simulink model "CtrPlatform"  (Simulink 7.9)
settings: Solver=ode3  StartTime=0.0  StopTime=8  FixedStep=Ts  RelTol=1e-3
InitFcn:
  | eval('CtrPlatformCfg')
StopFcn:
  | eval('CtrPlotTrj')
values from neighbouring files (symbols this model uses):
  A = [a1 a2 a3 a4 a5 a6]/180*pi    [Config.m]    (also in CtrPlatformCfg.m)
  a2 = 0    [Config.m]    (also in CtrPlatformCfg.m)
  a3 = 0    [Config.m]    (also in CtrPlatformCfg.m)
  a4 = 0    [Config.m]    (also in CtrPlatformCfg.m)
  a5 = 90    [Config.m]    (also in CtrPlatformCfg.m)
  a6 = 0    [Config.m]    (also in CtrPlatformCfg.m)
  Cen = Cen(:)'    [Config.m]    (also in CtrPlatformCfg.m; DynEulerTest.m = Cen'; EfDynCAD.m = [cen1,cen2,cen3,cen4,cen5,cen6]')
  CurPulseFreq = 0.25*2*pi    (= 1.57079632679)    [Config.m]    (also in CtrPlatformCfg.m)
  Deg2Rad = pi/180    (= 0.0174532925199)    [Config.m]    (also in CtrPlatformCfg.m)
  DisturbSelect = 2    [Config.m]    (also in CtrPlatformCfg.m)
  DynTrjMode = 3    [Config.m]    (also in CtrPlatformCfg.m = 1)
  FbDisturbSelect = 2    [Config.m]    (also in CtrPlatformCfg.m)
  freq = tvel/radius    (= 1)    [Config.m]    (also in CtrPlatformCfg.m)
  FrictionSelect = 2    [CtrPlatformCfg.m]
  Gravity = 9.8    [Config.m]    (also in CtrPlatformCfg.m)
  Ie1 = in1(:)'    [Config.m]    (also in CtrPlatformCfg.m; DynEulerTest.m = in1(:); EfDynCAD.m = in1(:))
  Ie2 = in2(:)'    [Config.m]    (also in CtrPlatformCfg.m; DynEulerTest.m = in2(:); EfDynCAD.m = in2(:))
  Ie3 = in3(:)'    [Config.m]    (also in CtrPlatformCfg.m; DynEulerTest.m = in3(:); EfDynCAD.m = in3(:))
  Ie4 = in4(:)'    [Config.m]    (also in CtrPlatformCfg.m; DynEulerTest.m = in4(:); EfDynCAD.m = in4(:))
  Ie5 = in5(:)'    [Config.m]    (also in CtrPlatformCfg.m; DynEulerTest.m = in5(:); EfDynCAD.m = in5(:))
  Ie6 = in6(:)'    [Config.m]    (also in CtrPlatformCfg.m; DynEulerTest.m = in6(:); EfDynCAD.m = in6(:))
  in1 = [5.2954 -0.2565 -0.6366;-0.2565 4.7000 0.2830;-0.6366 0.2829 5.8635]    [Config.m]    (also in CtrPlatformCfg.m; DynEulerTest.m; EfDynCAD.m = [0.54  -0.01 0.23)
  in2 = [5.8840 0.0072 0.0135;0.0072 6.0178 -0.1907;0.0135 -0.1907 0.3374]    [Config.m]    (also in CtrPlatformCfg.m; DynEulerTest.m; EfDynCAD.m = (R_x*R_z)*in2*(R_x*R_z)')
  in3 = [1.8201 -0.2274 -0.3112;-0.2274 2.2537 -0.1441;-0.3112 -0.1441 1.9485]    [Config.m]    (also in CtrPlatformCfg.m; DynEulerTest.m; EfDynCAD.m = (R_x*R_z)*in3*(R_x*R_z)')
  in4 = [0.0607 -0.0922 0;-0.0922 1.4493 0;0 0 1.4620]    [Config.m]    (also in CtrPlatformCfg.m; DynEulerTest.m = [0.0607 -0.0922 0;-0.0922 1.4493 0;0 0,1.4620]; EfDynCAD.m = (R_y*Rz)*in4*(R_y*Rz)')
  in5 = [0.0191 0.0032 0;0.0032 0.0228 0;0 0 0.0291]    [Config.m]    (also in CtrPlatformCfg.m; DynEulerTest.m; EfDynCAD.m = (R_x*R_y)*in5*(R_x*R_y)')
  in6 = [0.0012 0 0;0 0.0007 0;0 0 0.0007]    [Config.m]    (also in CtrPlatformCfg.m; DynEulerTest.m; EfDynCAD.m = (R_y*Rz)*in6*(R_y*Rz)')
  init_Endx = gd_init(1,4)    [Config.m]    (also in CtrPlatformCfg.m)
  init_Endy = gd_init(2,4)    [Config.m]    (also in CtrPlatformCfg.m)
  init_Endz = gd_init(3,4)    [Config.m]    (also in CtrPlatformCfg.m)
  init_Rot = gd_init(1:3,1:3)    [Config.m]    (also in CtrPlatformCfg.m)
  JntOffset1 = A(1)    [Config.m]    (also in CtrPlatformCfg.m)
  JntOffset2 = A(2)    [Config.m]    (also in CtrPlatformCfg.m)
  JntOffset3 = A(3)    [Config.m]    (also in CtrPlatformCfg.m)
  JntOffset4 = A(4)    [Config.m]    (also in CtrPlatformCfg.m)
  JntOffset5 = A(5)    [Config.m]    (also in CtrPlatformCfg.m)
  JntOffset6 = A(6)    [Config.m]    (also in CtrPlatformCfg.m)
  L = [l1 l2 l3 l4 l5 l6 l7 l8 l9]    [Config.m]    (also in CtrPlatformCfg.m)
  LinePTs2RadpS = 2*pi/(EncRes*Ts)./Gear    [Config.m]    (also in CtrPlatformCfg.m)
  LinePTs2Rpm = 60/(EncRes*Ts)    (= 7.32421875)    [Config.m]    (also in CtrPlatformCfg.m)
  Ma = [ma1 ma2 ma3 ma4 ma5 ma6]    [Config.m]    (also in CtrPlatformCfg.m; DynEulerTest.m = [ma1; ma2; ma3; ma4; ma5; ma6]; EfDynCAD.m = [ma1 ma2 ma3 ma4 ma5 ma6]')
  ma1 = 170.31    [Config.m]    (also in CtrPlatformCfg.m; DynEulerTest.m; EfDynCAD.m = 77.75)
  ma2 = 63.74    [Config.m]    (also in CtrPlatformCfg.m; DynEulerTest.m; EfDynCAD.m = 32.31)
  ma3 = 98.98    [Config.m]    (also in CtrPlatformCfg.m; DynEulerTest.m; EfDynCAD.m = 18.61)
  ma4 = 24.46    [Config.m]    (also in CtrPlatformCfg.m; DynEulerTest.m; EfDynCAD.m = 15.65)
  ma5 = 5.24    [Config.m]    (also in CtrPlatformCfg.m; DynEulerTest.m; EfDynCAD.m = 3.32)
  ma6 = 0.6    [Config.m]    (also in CtrPlatformCfg.m; DynEulerTest.m; EfDynCAD.m)
  PosPulseEnable = 1    [Config.m]    (also in CtrPlatformCfg.m)
  PosVelPulseGain = 500    [Config.m]    (also in CtrPlatformCfg.m)
  Rad2Line = Gear*EncRes/(2*pi)    [Config.m]    (also in CtrPlatformCfg.m)
  Rpm2LinePTs = EncRes*Ts/60    (= 0.136533333333)    [Config.m]    (also in CtrPlatformCfg.m)
  TrajSwitch = 1    [Config.m]    (also in CtrPlatformCfg.m)
  Trq2Cur = Trq2Cur./Cur2Trq    [Config.m]    (also in CtrPlatformCfg.m)
  Ts = 1/FrHz    (= 0.00025)    [Config.m]    (also in CtrPlatformCfg.m)
  Ts_Dyn = Ts    (= 0.00025)    [Config.m]    (also in CtrPlatformCfg.m)
  tvel = 120    [Config.m]    (also in CtrPlatformCfg.m)
  VelLpAxisNum = 1    [Config.m]    (also in CtrPlatformCfg.m)
  VelPulseEnable = 0    [Config.m]    (also in CtrPlatformCfg.m)
  VelPulseGain = 500    [Config.m]    (also in CtrPlatformCfg.m)
  Volt2Trq = Volt2Trq./Trq2Cur    [Config.m]    (also in CtrPlatformCfg.m)
undefined symbols (not defined in the file or in its folder): a1, DiscIntNeverNeededParam, RobotAxis
libraries: simulink x85, mblibv1 x35, powerlib_extras x25, commnoisgen2 x2
(part 3 of 5)

== system CtrPlatform/Trajectory Generator/Circle in Descartes Space ==
  Difference{,1..3} (4 alike) : simulink/Discrete/Difference  ICPrevInput=0.0  InputProcessing=Inherited  OutMin=[]  OutMax=[]  OutDataType=fixdt(1, 16)  OutScaling=2^-10  DoSatur=off
  Discrete-Time Integrator : DiscreteIntegrator  InitialCondition=init_Endx  SampleTime=Ts_Dyn  ICPrevOutput=DiscIntNeverNeededParam  ICPrevScaledInput=DiscIntNeverNeededParam
  Discrete-Time Integrator1 : DiscreteIntegrator  InitialCondition=init_Endy  SampleTime=Ts_Dyn  ICPrevOutput=DiscIntNeverNeededParam  ICPrevScaledInput=DiscIntNeverNeededParam
  Discrete-Time Integrator2 : DiscreteIntegrator  InitialCondition=init_Endz  SampleTime=Ts_Dyn  ICPrevOutput=DiscIntNeverNeededParam  ICPrevScaledInput=DiscIntNeverNeededParam
  EndVelocity : Subsystem
  Inverse Kinematic : MATLAB Function  TreatAsAtomicUnit=on
  Jacobian : MATLAB Function  TreatAsAtomicUnit=on
  Mux{1..3,5..6} (5 alike) : Mux  Inputs=3
  Mux4 : Mux  Inputs=5
  Rad2Deg : Gain  Gain=180/pi
  "Re-group " : Subsystem
  Zero : Gain  Gain=0
  Zero1 : Gain  Gain=1/Ts_Dyn
  Zero2 : Gain  Gain=1/Ts_Dyn
  Ref_JJVVAA : Outport
  RefEnd : Outport  Port=2
  Ref_JVAJVA : Outport  Port=3
  wires:
  Discrete-Time Integrator/1 -> Mux2/1
  Discrete-Time Integrator1/1 -> Mux2/2
  EndVelocity/1(EndVx) -> Mux1/1, Mux5/1, Difference/1, Discrete-Time Integrator/1
  EndVelocity/2(EndVy) -> Mux1/2, Mux5/2, Difference1/1, Discrete-Time Integrator1/1
  EndVelocity/3(EndVz) -> Mux1/3, Mux5/3, Difference2/1, Discrete-Time Integrator2/1
  Discrete-Time Integrator2/1 -> Mux2/3
  Mux2/1 -> Inverse Kinematic/1(EndPos), Mux4/1
  Inverse Kinematic/1(Theta) -> Jacobian/1(Theta), Mux3/1
  Mux4/1 -> RefEnd/1
  Difference/1 -> Mux6/1
  Difference1/1 -> Mux6/2
  Difference2/1 -> Mux6/3
  Mux1/1 -> Jacobian/2(EndVel)
  Jacobian/1(Omega) -> Mux3/2, Difference3/1
  Difference3/1 -> Zero2/1
  Mux3/1 -> Ref_JJVVAA/1, "Re-group "/1(JJVVAA)
  "Re-group "/1(JVAJVA) -> Rad2Deg/1
  Mux5/1 -> Mux4/2
  Mux6/1 -> Zero1/1
  Zero/1 -> Mux4/3, Mux4/5
  Rad2Deg/1 -> Ref_JVAJVA/1
  Zero1/1 -> Mux4/4, Zero/1
  Zero2/1 -> Mux3/3

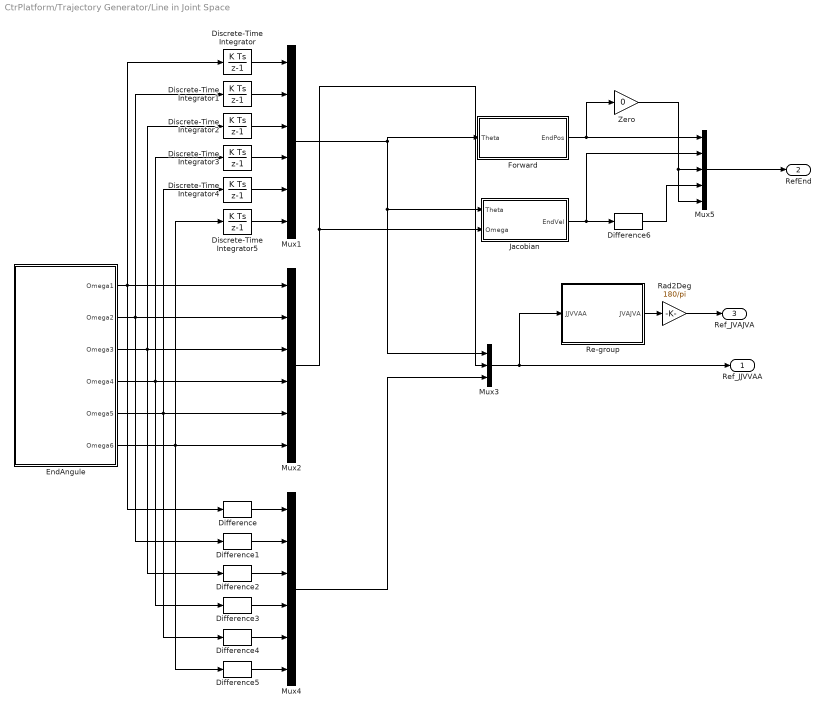
== system CtrPlatform/Trajectory Generator/Line in Joint Space ==
  Difference{,1..6} (7 alike) : simulink/Discrete/Difference  ICPrevInput=0.0  InputProcessing=Inherited  OutMin=[]  OutMax=[]  OutDataType=fixdt(1, 16)  OutScaling=2^-10  DoSatur=off
  Discrete-Time Integrator : DiscreteIntegrator  InitialCondition=a1/180*pi  SampleTime=Ts_Dyn  ICPrevOutput=DiscIntNeverNeededParam  ICPrevScaledInput=DiscIntNeverNeededParam
  Discrete-Time Integrator1 : DiscreteIntegrator  InitialCondition=a2/180*pi  SampleTime=Ts_Dyn  ICPrevOutput=DiscIntNeverNeededParam  ICPrevScaledInput=DiscIntNeverNeededParam
  Discrete-Time Integrator2 : DiscreteIntegrator  InitialCondition=a3/180*pi  SampleTime=Ts_Dyn  ICPrevOutput=DiscIntNeverNeededParam  ICPrevScaledInput=DiscIntNeverNeededParam
  Discrete-Time Integrator3 : DiscreteIntegrator  InitialCondition=a4/180*pi  SampleTime=Ts_Dyn  ICPrevOutput=DiscIntNeverNeededParam  ICPrevScaledInput=DiscIntNeverNeededParam
  Discrete-Time Integrator4 : DiscreteIntegrator  InitialCondition=a5/180*pi  SampleTime=Ts_Dyn  ICPrevOutput=DiscIntNeverNeededParam  ICPrevScaledInput=DiscIntNeverNeededParam
  Discrete-Time Integrator5 : DiscreteIntegrator  InitialCondition=a6/180*pi  SampleTime=Ts_Dyn  ICPrevOutput=DiscIntNeverNeededParam  ICPrevScaledInput=DiscIntNeverNeededParam
  EndAngule : Subsystem
  Forward : MATLAB Function  TreatAsAtomicUnit=on
  Jacobian : MATLAB Function  TreatAsAtomicUnit=on
  Mux1 : Mux  Inputs=6
  Mux2 : Mux  Inputs=6
  Mux3 : Mux  Inputs=3
  Mux4 : Mux  Inputs=6
  Mux5 : Mux  Inputs=5
  Rad2Deg : Gain  Gain=180/pi
  "Re-group " : Subsystem
  Zero : Gain  Gain=0
  Ref_JJVVAA : Outport
  RefEnd : Outport  Port=2
  Ref_JVAJVA : Outport  Port=3
  wires:
  Forward/1(EndPos) -> Mux5/1, Zero/1
  Mux5/1 -> RefEnd/1
  Mux4/1 -> Mux3/3
  Mux1/1 -> Jacobian/1(Theta), Mux3/1, Forward/1(Theta)
  Mux2/1 -> Jacobian/2(Omega), Mux3/2
  Difference5/1 -> Mux4/6
  Difference4/1 -> Mux4/5
  Difference3/1 -> Mux4/4
  Difference2/1 -> Mux4/3
  Difference1/1 -> Mux4/2
  Difference/1 -> Mux4/1
  Discrete-Time Integrator5/1 -> Mux1/6
  Discrete-Time Integrator4/1 -> Mux1/5
  Discrete-Time Integrator3/1 -> Mux1/4
  Discrete-Time Integrator2/1 -> Mux1/3
  Discrete-Time Integrator1/1 -> Mux1/2
  Discrete-Time Integrator/1 -> Mux1/1
  EndAngule/6(Omega6) -> Mux2/6, Discrete-Time Integrator5/1, Difference5/1
  EndAngule/5(Omega5) -> Mux2/5, Discrete-Time Integrator4/1, Difference4/1
  EndAngule/4(Omega4) -> Mux2/4, Discrete-Time Integrator3/1, Difference3/1
  EndAngule/3(Omega3) -> Mux2/3, Discrete-Time Integrator2/1, Difference2/1
  EndAngule/2(Omega2) -> Mux2/2, Discrete-Time Integrator1/1, Difference1/1
  EndAngule/1(Omega1) -> Mux2/1, Discrete-Time Integrator/1, Difference/1
  Mux3/1 -> Ref_JJVVAA/1, "Re-group "/1(JJVVAA)
  "Re-group "/1(JVAJVA) -> Rad2Deg/1
  Jacobian/1(EndVel) -> Mux5/2, Difference6/1
  Difference6/1 -> Mux5/4
  Zero/1 -> Mux5/3, Mux5/5
  Rad2Deg/1 -> Ref_JVAJVA/1

== system CtrPlatform/Trajectory Generator/Still ==
  Difference{,1..3} (4 alike) : simulink/Discrete/Difference  ICPrevInput=0.0  InputProcessing=Inherited  OutMin=[]  OutMax=[]  OutDataType=fixdt(1, 16)  OutScaling=2^-10  DoSatur=off
  Discrete-Time Integrator : DiscreteIntegrator  InitialCondition=init_Endx  SampleTime=Ts_Dyn  ICPrevOutput=DiscIntNeverNeededParam  ICPrevScaledInput=DiscIntNeverNeededParam
  Discrete-Time Integrator1 : DiscreteIntegrator  InitialCondition=init_Endy  SampleTime=Ts_Dyn  ICPrevOutput=DiscIntNeverNeededParam  ICPrevScaledInput=DiscIntNeverNeededParam
  Discrete-Time Integrator2 : DiscreteIntegrator  InitialCondition=init_Endz  SampleTime=Ts_Dyn  ICPrevOutput=DiscIntNeverNeededParam  ICPrevScaledInput=DiscIntNeverNeededParam
  EndVelocity : Subsystem
  Inverse Kinematic : MATLAB Function  TreatAsAtomicUnit=on
  Jacobian : MATLAB Function  TreatAsAtomicUnit=on
  Mux{1..3,5..6} (5 alike) : Mux  Inputs=3
  Mux4 : Mux  Inputs=5
  Rad2Deg : Gain  Gain=180/pi
  "Re-group " : Subsystem
  Zero : Gain  Gain=0
  Ref_JJVVAA : Outport
  RefEnd : Outport  Port=2
  Ref_JVAJVA : Outport  Port=3
  wires:
  Zero/1 -> Mux4/5, Mux4/3
  Mux6/1 -> Zero/1, Mux4/4
  Mux5/1 -> Mux4/2
  "Re-group "/1(JVAJVA) -> Rad2Deg/1
  Mux3/1 -> "Re-group "/1(JJVVAA), Ref_JJVVAA/1
  Difference3/1 -> Mux3/3
  Jacobian/1(Omega) -> Mux3/2, Difference3/1
  Mux1/1 -> Jacobian/2(EndVel)
  Difference2/1 -> Mux6/3
  Difference1/1 -> Mux6/2
  Difference/1 -> Mux6/1
  Mux4/1 -> RefEnd/1
  Inverse Kinematic/1(Theta) -> Mux3/1, Jacobian/1(Theta)
  Mux2/1 -> Mux4/1, Inverse Kinematic/1(EndPos)
  Discrete-Time Integrator2/1 -> Mux2/3
  EndVelocity/3(EndVz) -> Mux5/3, Difference2/1, Mux1/3, Discrete-Time Integrator2/1
  EndVelocity/2(EndVy) -> Mux5/2, Difference1/1, Mux1/2, Discrete-Time Integrator1/1
  EndVelocity/1(EndVx) -> Mux5/1, Difference/1, Mux1/1, Discrete-Time Integrator/1
  Discrete-Time Integrator1/1 -> Mux2/2
  Discrete-Time Integrator/1 -> Mux2/1
  Rad2Deg/1 -> Ref_JVAJVA/1

== system CtrPlatform/Controller/Controller Axis 1/EncDiff2Vel(LpTs) ==
  Enc : Inport
  Add : Sum  Inputs=+-
  Discrete  2nd-Order Filter : powerlib_extras/Discrete  Control Blocks/Discrete  2nd-Order Filter  FilterType=Lowpass  Fo=200  Zeta=0.707  Ts=Ts  Initialize=off  Vac_Init=[0.8 -25 60]  Vdc_Init=-0.4  PlotResponse=off  param1=[1 5000 10]
  EncVel(rpm) : Scope
      settings: SaveName=ScopeData33
  Integer Delay : Delay  DelayLength=1  InitialCondition=0  InputProcessing=Inherited
  LinePTs2Rpm : Gain  Gain=LinePTs2Rpm
  Vel : Outport
  wires:
  LinePTs2Rpm/1 -> EncVel(rpm)/1
  Integer Delay/1 -> Add/2
  Enc/1 -> Add/1, Integer Delay/1
  Discrete  2nd-Order Filter/1 -> LinePTs2Rpm/1, Vel/1
  Add/1 -> Discrete  2nd-Order Filter/1

== system CtrPlatform/Controller/Controller Axis 1/EncDiff2Vel(LpTs)1 ==
  Enc : Inport
  Add : Sum  Inputs=+-
  Discrete  2nd-Order Filter : powerlib_extras/Discrete  Control Blocks/Discrete  2nd-Order Filter  FilterType=Lowpass  Fo=200  Zeta=0.707  Ts=Ts  Initialize=off  Vac_Init=[0.8 -25 60]  Vdc_Init=-0.4  PlotResponse=off  param1=[1 5000 10]
  EncVel(rpm) : Scope
      settings: SaveName=ScopeData33
  Integer Delay : Delay  DelayLength=1  InitialCondition=0  InputProcessing=Inherited
  LinePTs2Rpm : Gain  Gain=LinePTs2Rpm
  Vel : Outport
  wires:
  Add/1 -> Discrete  2nd-Order Filter/1
  Discrete  2nd-Order Filter/1 -> Vel/1, LinePTs2Rpm/1
  Enc/1 -> Integer Delay/1, Add/1
  Integer Delay/1 -> Add/2
  LinePTs2Rpm/1 -> EncVel(rpm)/1

== system CtrPlatform/Controller/Controller Axis 1/Error Check and Lock Error ==
  PositionCheck(Line) : Inport
  VelocityCheck(LpTs) : Inport  Port=2
  Abs : Abs
  Abs1 : Abs
  Compare To Constant : simulink/Logic and Bit Operations/Compare To Constant  relop=<=  const=VelErrorCheckLimit  OutDataTypeStr=uint8  ZeroCross=off
  Compare To Constant1 : simulink/Logic and Bit Operations/Compare To Constant  relop=<=  const=PosErrorCheckLimit  OutDataTypeStr=uint8  ZeroCross=off
  Logical Operator : Logic  Inputs=3  AllPortsSameDT=off  OutDataTypeStr=boolean
  Unit Delay : UnitDelay  X0=1  SampleTime=Ts
  ErrorFlag : Outport
  wires:
  Logical Operator/1 -> Unit Delay/1, ErrorFlag/1
  Compare To Constant/1 -> Logical Operator/2
  Compare To Constant1/1 -> Logical Operator/1
  Abs1/1 -> Compare To Constant1/1
  Abs/1 -> Compare To Constant/1
  Unit Delay/1 -> Logical Operator/3
  PositionCheck(Line)/1 -> Abs1/1
  VelocityCheck(LpTs)/1 -> Abs/1

== system CtrPlatform/Controller/Controller Axis 1/IncPos(Line) ==
  Pos : Inport
  Add : Sum  Inputs=+-
  Int : DiscreteTransferFcn  Numerator=[1 0]  Denominator=[1 -1]  SampleTime=Ts
  Integer Delay : Delay  DelayLength=1  InitialCondition=InitialPos  InputProcessing=Inherited
  IncPos : Outport
  wires:
  Add/1 -> Int/1
  Pos/1 -> Add/1, Integer Delay/1
  Int/1 -> IncPos/1
  Integer Delay/1 -> Add/2

== system CtrPlatform/Controller/Controller Axis 1/Pos Controller ==
  Error(Line) : Inport
  Add1 : Sum  Inputs=+++
  D : Gain  Gain=Kd
  Diff : simulink/Discrete/Difference  ICPrevInput=0.0  InputProcessing=Inherited  OutMin=[]  OutMax=[]  OutDataType=sfix(16)  OutScaling=2^-10  DoSatur=off
  Discrete-Time Integrator : DiscreteIntegrator  SampleTime=Ts  ICPrevOutput=DiscIntNeverNeededParam  ICPrevScaledInput=DiscIntNeverNeededParam
  I : Gain  Gain=Ki
  p : Gain  Gain=Kp
  Vcmd(LpTs) : Outport
  wires:
  Diff/1 -> Add1/3
  Discrete-Time Integrator/1 -> Add1/2
  Add1/1 -> Vcmd(LpTs)/1
  Error(Line)/1 -> p/1, I/1, D/1
  p/1 -> Add1/1
  I/1 -> Discrete-Time Integrator/1
  D/1 -> Diff/1

== system CtrPlatform/Controller/Controller Axis 1/Vel Controller ==
  Error(LpTs) : Inport
  Add1 : Sum  Inputs=+++
  D : Gain  Gain=Kd
  Diff : simulink/Discrete/Difference  ICPrevInput=0.0  InputProcessing=Inherited  OutMin=[]  OutMax=[]  OutDataType=sfix(16)  OutScaling=2^-10  DoSatur=off
  Discrete-Time Integrator : DiscreteIntegrator  SampleTime=Ts  ICPrevOutput=DiscIntNeverNeededParam  ICPrevScaledInput=DiscIntNeverNeededParam
  I : Gain  Gain=Ki
  p : Gain  Gain=Kp
  Curcmd(Amp) : Outport
  wires:
  Discrete-Time Integrator/1 -> Add1/2
  Diff/1 -> Add1/3
  D/1 -> Diff/1
  Add1/1 -> Curcmd(Amp)/1
  I/1 -> Discrete-Time Integrator/1
  p/1 -> Add1/1
  Error(LpTs)/1 -> D/1, I/1, p/1

== system CtrPlatform/Controller/Controller Axis 2/EncDiff2Vel(LpTs) ==
  Enc : Inport
  Add : Sum  Inputs=+-
  Discrete  2nd-Order Filter : powerlib_extras/Discrete  Control Blocks/Discrete  2nd-Order Filter  FilterType=Lowpass  Fo=200  Zeta=0.707  Ts=Ts  Initialize=off  Vac_Init=[0.8 -25 60]  Vdc_Init=-0.4  PlotResponse=off  param1=[1 5000 10]
  EncVel(rpm) : Scope
      settings: SaveName=ScopeData33
  Integer Delay : Delay  DelayLength=1  InitialCondition=0  InputProcessing=Inherited
  LinePTs2Rpm : Gain  Gain=LinePTs2Rpm
  Vel : Outport
  wires:
  LinePTs2Rpm/1 -> EncVel(rpm)/1
  Integer Delay/1 -> Add/2
  Enc/1 -> Add/1, Integer Delay/1
  Discrete  2nd-Order Filter/1 -> LinePTs2Rpm/1, Vel/1
  Add/1 -> Discrete  2nd-Order Filter/1

== system CtrPlatform/Controller/Controller Axis 2/EncDiff2Vel(LpTs)1 ==
  Enc : Inport
  Add : Sum  Inputs=+-
  Discrete  2nd-Order Filter : powerlib_extras/Discrete  Control Blocks/Discrete  2nd-Order Filter  FilterType=Lowpass  Fo=200  Zeta=0.707  Ts=Ts  Initialize=off  Vac_Init=[0.8 -25 60]  Vdc_Init=-0.4  PlotResponse=off  param1=[1 5000 10]
  EncVel(rpm) : Scope
      settings: SaveName=ScopeData33
  Integer Delay : Delay  DelayLength=1  InitialCondition=0  InputProcessing=Inherited
  LinePTs2Rpm : Gain  Gain=LinePTs2Rpm
  Vel : Outport
  wires:
  Add/1 -> Discrete  2nd-Order Filter/1
  Discrete  2nd-Order Filter/1 -> Vel/1, LinePTs2Rpm/1
  Enc/1 -> Integer Delay/1, Add/1
  Integer Delay/1 -> Add/2
  LinePTs2Rpm/1 -> EncVel(rpm)/1

== system CtrPlatform/Controller/Controller Axis 2/Error Check and Lock Error ==
  PositionCheck(Line) : Inport
  VelocityCheck(LpTs) : Inport  Port=2
  Abs : Abs
  Abs1 : Abs
  Compare To Constant : simulink/Logic and Bit Operations/Compare To Constant  relop=<=  const=VelErrorCheckLimit  OutDataTypeStr=uint8  ZeroCross=off
  Compare To Constant1 : simulink/Logic and Bit Operations/Compare To Constant  relop=<=  const=PosErrorCheckLimit  OutDataTypeStr=uint8  ZeroCross=off
  Logical Operator : Logic  Inputs=3  AllPortsSameDT=off  OutDataTypeStr=boolean
  Unit Delay : UnitDelay  X0=1  SampleTime=Ts
  ErrorFlag : Outport
  wires:
  Logical Operator/1 -> Unit Delay/1, ErrorFlag/1
  Compare To Constant/1 -> Logical Operator/2
  Compare To Constant1/1 -> Logical Operator/1
  Abs1/1 -> Compare To Constant1/1
  Abs/1 -> Compare To Constant/1
  Unit Delay/1 -> Logical Operator/3
  PositionCheck(Line)/1 -> Abs1/1
  VelocityCheck(LpTs)/1 -> Abs/1

== system CtrPlatform/Controller/Controller Axis 2/IncPos(Line) ==
  Pos : Inport
  Add : Sum  Inputs=+-
  Int : DiscreteTransferFcn  Numerator=[1 0]  Denominator=[1 -1]  SampleTime=Ts
  Integer Delay : Delay  DelayLength=1  InitialCondition=InitialPos  InputProcessing=Inherited
  IncPos : Outport
  wires:
  Add/1 -> Int/1
  Pos/1 -> Add/1, Integer Delay/1
  Int/1 -> IncPos/1
  Integer Delay/1 -> Add/2

== system CtrPlatform/Controller/Controller Axis 2/Pos Controller ==
  Error(Line) : Inport
  Add1 : Sum  Inputs=+++
  D : Gain  Gain=Kd
  Diff : simulink/Discrete/Difference  ICPrevInput=0.0  InputProcessing=Inherited  OutMin=[]  OutMax=[]  OutDataType=sfix(16)  OutScaling=2^-10  DoSatur=off
  Discrete-Time Integrator : DiscreteIntegrator  SampleTime=Ts  ICPrevOutput=DiscIntNeverNeededParam  ICPrevScaledInput=DiscIntNeverNeededParam
  I : Gain  Gain=Ki
  p : Gain  Gain=Kp
  Vcmd(LpTs) : Outport
  wires:
  Diff/1 -> Add1/3
  Discrete-Time Integrator/1 -> Add1/2
  Add1/1 -> Vcmd(LpTs)/1
  Error(Line)/1 -> p/1, I/1, D/1
  p/1 -> Add1/1
  I/1 -> Discrete-Time Integrator/1
  D/1 -> Diff/1

== system CtrPlatform/Controller/Controller Axis 2/Vel Controller ==
  Error(LpTs) : Inport
  Add1 : Sum  Inputs=+++
  D : Gain  Gain=Kd
  Diff : simulink/Discrete/Difference  ICPrevInput=0.0  InputProcessing=Inherited  OutMin=[]  OutMax=[]  OutDataType=sfix(16)  OutScaling=2^-10  DoSatur=off
  Discrete-Time Integrator : DiscreteIntegrator  SampleTime=Ts  ICPrevOutput=DiscIntNeverNeededParam  ICPrevScaledInput=DiscIntNeverNeededParam
  I : Gain  Gain=Ki
  p : Gain  Gain=Kp
  Curcmd(Amp) : Outport
  wires:
  Discrete-Time Integrator/1 -> Add1/2
  Diff/1 -> Add1/3
  D/1 -> Diff/1
  Add1/1 -> Curcmd(Amp)/1
  I/1 -> Discrete-Time Integrator/1
  p/1 -> Add1/1
  Error(LpTs)/1 -> D/1, I/1, p/1

== system CtrPlatform/Controller/Controller Axis 3/EncDiff2Vel(LpTs) ==
  Enc : Inport
  Add : Sum  Inputs=+-
  Discrete  2nd-Order Filter : powerlib_extras/Discrete  Control Blocks/Discrete  2nd-Order Filter  FilterType=Lowpass  Fo=200  Zeta=0.707  Ts=Ts  Initialize=off  Vac_Init=[0.8 -25 60]  Vdc_Init=-0.4  PlotResponse=off  param1=[1 5000 10]
  EncVel(rpm) : Scope
      settings: SaveName=ScopeData33
  Integer Delay : Delay  DelayLength=1  InitialCondition=0  InputProcessing=Inherited
  LinePTs2Rpm : Gain  Gain=LinePTs2Rpm
  Vel : Outport
  wires:
  LinePTs2Rpm/1 -> EncVel(rpm)/1
  Integer Delay/1 -> Add/2
  Enc/1 -> Add/1, Integer Delay/1
  Discrete  2nd-Order Filter/1 -> LinePTs2Rpm/1, Vel/1
  Add/1 -> Discrete  2nd-Order Filter/1

== system CtrPlatform/Controller/Controller Axis 3/EncDiff2Vel(LpTs)1 ==
  Enc : Inport
  Add : Sum  Inputs=+-
  Discrete  2nd-Order Filter : powerlib_extras/Discrete  Control Blocks/Discrete  2nd-Order Filter  FilterType=Lowpass  Fo=200  Zeta=0.707  Ts=Ts  Initialize=off  Vac_Init=[0.8 -25 60]  Vdc_Init=-0.4  PlotResponse=off  param1=[1 5000 10]
  EncVel(rpm) : Scope
      settings: SaveName=ScopeData33
  Integer Delay : Delay  DelayLength=1  InitialCondition=0  InputProcessing=Inherited
  LinePTs2Rpm : Gain  Gain=LinePTs2Rpm
  Vel : Outport
  wires:
  Add/1 -> Discrete  2nd-Order Filter/1
  Discrete  2nd-Order Filter/1 -> Vel/1, LinePTs2Rpm/1
  Enc/1 -> Integer Delay/1, Add/1
  Integer Delay/1 -> Add/2
  LinePTs2Rpm/1 -> EncVel(rpm)/1

== system CtrPlatform/Controller/Controller Axis 3/Error Check and Lock Error ==
  PositionCheck(Line) : Inport
  VelocityCheck(LpTs) : Inport  Port=2
  Abs : Abs
  Abs1 : Abs
  Compare To Constant : simulink/Logic and Bit Operations/Compare To Constant  relop=<=  const=VelErrorCheckLimit  OutDataTypeStr=uint8  ZeroCross=off
  Compare To Constant1 : simulink/Logic and Bit Operations/Compare To Constant  relop=<=  const=PosErrorCheckLimit  OutDataTypeStr=uint8  ZeroCross=off
  Logical Operator : Logic  Inputs=3  AllPortsSameDT=off  OutDataTypeStr=boolean
  Unit Delay : UnitDelay  X0=1  SampleTime=Ts
  ErrorFlag : Outport
  wires:
  Logical Operator/1 -> Unit Delay/1, ErrorFlag/1
  Compare To Constant/1 -> Logical Operator/2
  Compare To Constant1/1 -> Logical Operator/1
  Abs1/1 -> Compare To Constant1/1
  Abs/1 -> Compare To Constant/1
  Unit Delay/1 -> Logical Operator/3
  PositionCheck(Line)/1 -> Abs1/1
  VelocityCheck(LpTs)/1 -> Abs/1

== system CtrPlatform/Controller/Controller Axis 3/IncPos(Line) ==
  Pos : Inport
  Add : Sum  Inputs=+-
  Int : DiscreteTransferFcn  Numerator=[1 0]  Denominator=[1 -1]  SampleTime=Ts
  Integer Delay : Delay  DelayLength=1  InitialCondition=InitialPos  InputProcessing=Inherited
  IncPos : Outport
  wires:
  Add/1 -> Int/1
  Pos/1 -> Add/1, Integer Delay/1
  Int/1 -> IncPos/1
  Integer Delay/1 -> Add/2

== system CtrPlatform/Controller/Controller Axis 3/Pos Controller ==
  Error(Line) : Inport
  Add1 : Sum  Inputs=+++
  D : Gain  Gain=Kd
  Diff : simulink/Discrete/Difference  ICPrevInput=0.0  InputProcessing=Inherited  OutMin=[]  OutMax=[]  OutDataType=sfix(16)  OutScaling=2^-10  DoSatur=off
  Discrete-Time Integrator : DiscreteIntegrator  SampleTime=Ts  ICPrevOutput=DiscIntNeverNeededParam  ICPrevScaledInput=DiscIntNeverNeededParam
  I : Gain  Gain=Ki
  p : Gain  Gain=Kp
  Vcmd(LpTs) : Outport
  wires:
  Diff/1 -> Add1/3
  Discrete-Time Integrator/1 -> Add1/2
  Add1/1 -> Vcmd(LpTs)/1
  Error(Line)/1 -> p/1, I/1, D/1
  p/1 -> Add1/1
  I/1 -> Discrete-Time Integrator/1
  D/1 -> Diff/1

== system CtrPlatform/Controller/Controller Axis 3/Vel Controller ==
  Error(LpTs) : Inport
  Add1 : Sum  Inputs=+++
  D : Gain  Gain=Kd
  Diff : simulink/Discrete/Difference  ICPrevInput=0.0  InputProcessing=Inherited  OutMin=[]  OutMax=[]  OutDataType=sfix(16)  OutScaling=2^-10  DoSatur=off
  Discrete-Time Integrator : DiscreteIntegrator  SampleTime=Ts  ICPrevOutput=DiscIntNeverNeededParam  ICPrevScaledInput=DiscIntNeverNeededParam
  I : Gain  Gain=Ki
  p : Gain  Gain=Kp
  Curcmd(Amp) : Outport
  wires:
  Discrete-Time Integrator/1 -> Add1/2
  Diff/1 -> Add1/3
  D/1 -> Diff/1
  Add1/1 -> Curcmd(Amp)/1
  I/1 -> Discrete-Time Integrator/1
  p/1 -> Add1/1
  Error(LpTs)/1 -> D/1, I/1, p/1

== system CtrPlatform/Controller/Controller Axis 4/EncDiff2Vel(LpTs) ==
  Enc : Inport
  Add : Sum  Inputs=+-
  Discrete  2nd-Order Filter : powerlib_extras/Discrete  Control Blocks/Discrete  2nd-Order Filter  FilterType=Lowpass  Fo=200  Zeta=0.707  Ts=Ts  Initialize=off  Vac_Init=[0.8 -25 60]  Vdc_Init=-0.4  PlotResponse=off  param1=[1 5000 10]
  EncVel(rpm) : Scope
      settings: SaveName=ScopeData33
  Integer Delay : Delay  DelayLength=1  InitialCondition=0  InputProcessing=Inherited
  LinePTs2Rpm : Gain  Gain=LinePTs2Rpm
  Vel : Outport
  wires:
  LinePTs2Rpm/1 -> EncVel(rpm)/1
  Integer Delay/1 -> Add/2
  Enc/1 -> Add/1, Integer Delay/1
  Discrete  2nd-Order Filter/1 -> LinePTs2Rpm/1, Vel/1
  Add/1 -> Discrete  2nd-Order Filter/1

== system CtrPlatform/Controller/Controller Axis 4/EncDiff2Vel(LpTs)1 ==
  Enc : Inport
  Add : Sum  Inputs=+-
  Discrete  2nd-Order Filter : powerlib_extras/Discrete  Control Blocks/Discrete  2nd-Order Filter  FilterType=Lowpass  Fo=200  Zeta=0.707  Ts=Ts  Initialize=off  Vac_Init=[0.8 -25 60]  Vdc_Init=-0.4  PlotResponse=off  param1=[1 5000 10]
  EncVel(rpm) : Scope
      settings: SaveName=ScopeData33
  Integer Delay : Delay  DelayLength=1  InitialCondition=0  InputProcessing=Inherited
  LinePTs2Rpm : Gain  Gain=LinePTs2Rpm
  Vel : Outport
  wires:
  Add/1 -> Discrete  2nd-Order Filter/1
  Discrete  2nd-Order Filter/1 -> Vel/1, LinePTs2Rpm/1
  Enc/1 -> Integer Delay/1, Add/1
  Integer Delay/1 -> Add/2
  LinePTs2Rpm/1 -> EncVel(rpm)/1

== system CtrPlatform/Controller/Controller Axis 4/Error Check and Lock Error ==
  PositionCheck(Line) : Inport
  VelocityCheck(LpTs) : Inport  Port=2
  Abs : Abs
  Abs1 : Abs
  Compare To Constant : simulink/Logic and Bit Operations/Compare To Constant  relop=<=  const=VelErrorCheckLimit  OutDataTypeStr=uint8  ZeroCross=off
  Compare To Constant1 : simulink/Logic and Bit Operations/Compare To Constant  relop=<=  const=PosErrorCheckLimit  OutDataTypeStr=uint8  ZeroCross=off
  Logical Operator : Logic  Inputs=3  AllPortsSameDT=off  OutDataTypeStr=boolean
  Unit Delay : UnitDelay  X0=1  SampleTime=Ts
  ErrorFlag : Outport
  wires:
  Logical Operator/1 -> Unit Delay/1, ErrorFlag/1
  Compare To Constant/1 -> Logical Operator/2
  Compare To Constant1/1 -> Logical Operator/1
  Abs1/1 -> Compare To Constant1/1
  Abs/1 -> Compare To Constant/1
  Unit Delay/1 -> Logical Operator/3
  PositionCheck(Line)/1 -> Abs1/1
  VelocityCheck(LpTs)/1 -> Abs/1

== system CtrPlatform/Controller/Controller Axis 4/IncPos(Line) ==
  Pos : Inport
  Add : Sum  Inputs=+-
  Int : DiscreteTransferFcn  Numerator=[1 0]  Denominator=[1 -1]  SampleTime=Ts
  Integer Delay : Delay  DelayLength=1  InitialCondition=InitialPos  InputProcessing=Inherited
  IncPos : Outport
  wires:
  Add/1 -> Int/1
  Pos/1 -> Add/1, Integer Delay/1
  Int/1 -> IncPos/1
  Integer Delay/1 -> Add/2

== system CtrPlatform/Controller/Controller Axis 4/Pos Controller ==
  Error(Line) : Inport
  Add1 : Sum  Inputs=+++
  D : Gain  Gain=Kd
  Diff : simulink/Discrete/Difference  ICPrevInput=0.0  InputProcessing=Inherited  OutMin=[]  OutMax=[]  OutDataType=sfix(16)  OutScaling=2^-10  DoSatur=off
  Discrete-Time Integrator : DiscreteIntegrator  SampleTime=Ts  ICPrevOutput=DiscIntNeverNeededParam  ICPrevScaledInput=DiscIntNeverNeededParam
  I : Gain  Gain=Ki
  p : Gain  Gain=Kp
  Vcmd(LpTs) : Outport
  wires:
  Diff/1 -> Add1/3
  Discrete-Time Integrator/1 -> Add1/2
  Add1/1 -> Vcmd(LpTs)/1
  Error(Line)/1 -> p/1, I/1, D/1
  p/1 -> Add1/1
  I/1 -> Discrete-Time Integrator/1
  D/1 -> Diff/1

== system CtrPlatform/Controller/Controller Axis 4/Vel Controller ==
  Error(LpTs) : Inport
  Add1 : Sum  Inputs=+++
  D : Gain  Gain=Kd
  Diff : simulink/Discrete/Difference  ICPrevInput=0.0  InputProcessing=Inherited  OutMin=[]  OutMax=[]  OutDataType=sfix(16)  OutScaling=2^-10  DoSatur=off
  Discrete-Time Integrator : DiscreteIntegrator  SampleTime=Ts  ICPrevOutput=DiscIntNeverNeededParam  ICPrevScaledInput=DiscIntNeverNeededParam
  I : Gain  Gain=Ki
  p : Gain  Gain=Kp
  Curcmd(Amp) : Outport
  wires:
  Discrete-Time Integrator/1 -> Add1/2
  Diff/1 -> Add1/3
  D/1 -> Diff/1
  Add1/1 -> Curcmd(Amp)/1
  I/1 -> Discrete-Time Integrator/1
  p/1 -> Add1/1
  Error(LpTs)/1 -> D/1, I/1, p/1

== system CtrPlatform/Controller/Controller Axis 5/EncDiff2Vel(LpTs) ==
  Enc : Inport
  Add : Sum  Inputs=+-
  Discrete  2nd-Order Filter : powerlib_extras/Discrete  Control Blocks/Discrete  2nd-Order Filter  FilterType=Lowpass  Fo=200  Zeta=0.707  Ts=Ts  Initialize=off  Vac_Init=[0.8 -25 60]  Vdc_Init=-0.4  PlotResponse=off  param1=[1 5000 10]
  EncVel(rpm) : Scope
      settings: SaveName=ScopeData33
  Integer Delay : Delay  DelayLength=1  InitialCondition=0  InputProcessing=Inherited
  LinePTs2Rpm : Gain  Gain=LinePTs2Rpm
  Vel : Outport
  wires:
  LinePTs2Rpm/1 -> EncVel(rpm)/1
  Integer Delay/1 -> Add/2
  Enc/1 -> Add/1, Integer Delay/1
  Discrete  2nd-Order Filter/1 -> LinePTs2Rpm/1, Vel/1
  Add/1 -> Discrete  2nd-Order Filter/1

== system CtrPlatform/Controller/Controller Axis 5/EncDiff2Vel(LpTs)1 ==
  Enc : Inport
  Add : Sum  Inputs=+-
  Discrete  2nd-Order Filter : powerlib_extras/Discrete  Control Blocks/Discrete  2nd-Order Filter  FilterType=Lowpass  Fo=200  Zeta=0.707  Ts=Ts  Initialize=off  Vac_Init=[0.8 -25 60]  Vdc_Init=-0.4  PlotResponse=off  param1=[1 5000 10]
  EncVel(rpm) : Scope
      settings: SaveName=ScopeData33
  Integer Delay : Delay  DelayLength=1  InitialCondition=0  InputProcessing=Inherited
  LinePTs2Rpm : Gain  Gain=LinePTs2Rpm
  Vel : Outport
  wires:
  Add/1 -> Discrete  2nd-Order Filter/1
  Discrete  2nd-Order Filter/1 -> Vel/1, LinePTs2Rpm/1
  Enc/1 -> Integer Delay/1, Add/1
  Integer Delay/1 -> Add/2
  LinePTs2Rpm/1 -> EncVel(rpm)/1

== system CtrPlatform/Controller/Controller Axis 5/Error Check and Lock Error ==
  PositionCheck(Line) : Inport
  VelocityCheck(LpTs) : Inport  Port=2
  Abs : Abs
  Abs1 : Abs
  Compare To Constant : simulink/Logic and Bit Operations/Compare To Constant  relop=<=  const=VelErrorCheckLimit  OutDataTypeStr=uint8  ZeroCross=off
  Compare To Constant1 : simulink/Logic and Bit Operations/Compare To Constant  relop=<=  const=PosErrorCheckLimit  OutDataTypeStr=uint8  ZeroCross=off
  Logical Operator : Logic  Inputs=3  AllPortsSameDT=off  OutDataTypeStr=boolean
  Unit Delay : UnitDelay  X0=1  SampleTime=Ts
  ErrorFlag : Outport
  wires:
  Logical Operator/1 -> Unit Delay/1, ErrorFlag/1
  Compare To Constant/1 -> Logical Operator/2
  Compare To Constant1/1 -> Logical Operator/1
  Abs1/1 -> Compare To Constant1/1
  Abs/1 -> Compare To Constant/1
  Unit Delay/1 -> Logical Operator/3
  PositionCheck(Line)/1 -> Abs1/1
  VelocityCheck(LpTs)/1 -> Abs/1

== system CtrPlatform/Controller/Controller Axis 5/IncPos(Line) ==
  Pos : Inport
  Add : Sum  Inputs=+-
  Int : DiscreteTransferFcn  Numerator=[1 0]  Denominator=[1 -1]  SampleTime=Ts
  Integer Delay : Delay  DelayLength=1  InitialCondition=InitialPos  InputProcessing=Inherited
  IncPos : Outport
  wires:
  Add/1 -> Int/1
  Pos/1 -> Add/1, Integer Delay/1
  Int/1 -> IncPos/1
  Integer Delay/1 -> Add/2

== system CtrPlatform/Controller/Controller Axis 5/Pos Controller ==
  Error(Line) : Inport
  Add1 : Sum  Inputs=+++
  D : Gain  Gain=Kd
  Diff : simulink/Discrete/Difference  ICPrevInput=0.0  InputProcessing=Inherited  OutMin=[]  OutMax=[]  OutDataType=sfix(16)  OutScaling=2^-10  DoSatur=off
  Discrete-Time Integrator : DiscreteIntegrator  SampleTime=Ts  ICPrevOutput=DiscIntNeverNeededParam  ICPrevScaledInput=DiscIntNeverNeededParam
  I : Gain  Gain=Ki
  p : Gain  Gain=Kp
  Vcmd(LpTs) : Outport
  wires:
  Diff/1 -> Add1/3
  Discrete-Time Integrator/1 -> Add1/2
  Add1/1 -> Vcmd(LpTs)/1
  Error(Line)/1 -> p/1, I/1, D/1
  p/1 -> Add1/1
  I/1 -> Discrete-Time Integrator/1
  D/1 -> Diff/1

== system CtrPlatform/Controller/Controller Axis 5/Vel Controller ==
  Error(LpTs) : Inport
  Add1 : Sum  Inputs=+++
  D : Gain  Gain=Kd
  Diff : simulink/Discrete/Difference  ICPrevInput=0.0  InputProcessing=Inherited  OutMin=[]  OutMax=[]  OutDataType=sfix(16)  OutScaling=2^-10  DoSatur=off
  Discrete-Time Integrator : DiscreteIntegrator  SampleTime=Ts  ICPrevOutput=DiscIntNeverNeededParam  ICPrevScaledInput=DiscIntNeverNeededParam
  I : Gain  Gain=Ki
  p : Gain  Gain=Kp
  Curcmd(Amp) : Outport
  wires:
  Discrete-Time Integrator/1 -> Add1/2
  Diff/1 -> Add1/3
  D/1 -> Diff/1
  Add1/1 -> Curcmd(Amp)/1
  I/1 -> Discrete-Time Integrator/1
  p/1 -> Add1/1
  Error(LpTs)/1 -> D/1, I/1, p/1

== system CtrPlatform/Controller/Controller Axis 6/EncDiff2Vel(LpTs) ==
  Enc : Inport
  Add : Sum  Inputs=+-
  Discrete  2nd-Order Filter : powerlib_extras/Discrete  Control Blocks/Discrete  2nd-Order Filter  FilterType=Lowpass  Fo=200  Zeta=0.707  Ts=Ts  Initialize=off  Vac_Init=[0.8 -25 60]  Vdc_Init=-0.4  PlotResponse=off  param1=[1 5000 10]
  EncVel(rpm) : Scope
      settings: SaveName=ScopeData33
  Integer Delay : Delay  DelayLength=1  InitialCondition=0  InputProcessing=Inherited
  LinePTs2Rpm : Gain  Gain=LinePTs2Rpm
  Vel : Outport
  wires:
  LinePTs2Rpm/1 -> EncVel(rpm)/1
  Integer Delay/1 -> Add/2
  Enc/1 -> Add/1, Integer Delay/1
  Discrete  2nd-Order Filter/1 -> LinePTs2Rpm/1, Vel/1
  Add/1 -> Discrete  2nd-Order Filter/1

== system CtrPlatform/Controller/Controller Axis 6/EncDiff2Vel(LpTs)1 ==
  Enc : Inport
  Add : Sum  Inputs=+-
  Discrete  2nd-Order Filter : powerlib_extras/Discrete  Control Blocks/Discrete  2nd-Order Filter  FilterType=Lowpass  Fo=200  Zeta=0.707  Ts=Ts  Initialize=off  Vac_Init=[0.8 -25 60]  Vdc_Init=-0.4  PlotResponse=off  param1=[1 5000 10]
  EncVel(rpm) : Scope
      settings: SaveName=ScopeData33
  Integer Delay : Delay  DelayLength=1  InitialCondition=0  InputProcessing=Inherited
  LinePTs2Rpm : Gain  Gain=LinePTs2Rpm
  Vel : Outport
  wires:
  Add/1 -> Discrete  2nd-Order Filter/1
  Discrete  2nd-Order Filter/1 -> Vel/1, LinePTs2Rpm/1
  Enc/1 -> Integer Delay/1, Add/1
  Integer Delay/1 -> Add/2
  LinePTs2Rpm/1 -> EncVel(rpm)/1

== system CtrPlatform/Controller/Controller Axis 6/Error Check and Lock Error ==
  PositionCheck(Line) : Inport
  VelocityCheck(LpTs) : Inport  Port=2
  Abs : Abs
  Abs1 : Abs
  Compare To Constant : simulink/Logic and Bit Operations/Compare To Constant  relop=<=  const=VelErrorCheckLimit  OutDataTypeStr=uint8  ZeroCross=off
  Compare To Constant1 : simulink/Logic and Bit Operations/Compare To Constant  relop=<=  const=PosErrorCheckLimit  OutDataTypeStr=uint8  ZeroCross=off
  Logical Operator : Logic  Inputs=3  AllPortsSameDT=off  OutDataTypeStr=boolean
  Unit Delay : UnitDelay  X0=1  SampleTime=Ts
  ErrorFlag : Outport
  wires:
  Logical Operator/1 -> Unit Delay/1, ErrorFlag/1
  Compare To Constant/1 -> Logical Operator/2
  Compare To Constant1/1 -> Logical Operator/1
  Abs1/1 -> Compare To Constant1/1
  Abs/1 -> Compare To Constant/1
  Unit Delay/1 -> Logical Operator/3
  PositionCheck(Line)/1 -> Abs1/1
  VelocityCheck(LpTs)/1 -> Abs/1

== system CtrPlatform/Controller/Controller Axis 6/IncPos(Line) ==
  Pos : Inport
  Add : Sum  Inputs=+-
  Int : DiscreteTransferFcn  Numerator=[1 0]  Denominator=[1 -1]  SampleTime=Ts
  Integer Delay : Delay  DelayLength=1  InitialCondition=InitialPos  InputProcessing=Inherited
  IncPos : Outport
  wires:
  Add/1 -> Int/1
  Pos/1 -> Add/1, Integer Delay/1
  Int/1 -> IncPos/1
  Integer Delay/1 -> Add/2

== system CtrPlatform/Controller/Controller Axis 6/Pos Controller ==
  Error(Line) : Inport
  Add1 : Sum  Inputs=+++
  D : Gain  Gain=Kd
  Diff : simulink/Discrete/Difference  ICPrevInput=0.0  InputProcessing=Inherited  OutMin=[]  OutMax=[]  OutDataType=sfix(16)  OutScaling=2^-10  DoSatur=off
  Discrete-Time Integrator : DiscreteIntegrator  SampleTime=Ts  ICPrevOutput=DiscIntNeverNeededParam  ICPrevScaledInput=DiscIntNeverNeededParam
  I : Gain  Gain=Ki
  p : Gain  Gain=Kp
  Vcmd(LpTs) : Outport
  wires:
  Diff/1 -> Add1/3
  Discrete-Time Integrator/1 -> Add1/2
  Add1/1 -> Vcmd(LpTs)/1
  Error(Line)/1 -> p/1, I/1, D/1
  p/1 -> Add1/1
  I/1 -> Discrete-Time Integrator/1
  D/1 -> Diff/1

== system CtrPlatform/Controller/Controller Axis 6/Vel Controller ==
  Error(LpTs) : Inport
  Add1 : Sum  Inputs=+++
  D : Gain  Gain=Kd
  Diff : simulink/Discrete/Difference  ICPrevInput=0.0  InputProcessing=Inherited  OutMin=[]  OutMax=[]  OutDataType=sfix(16)  OutScaling=2^-10  DoSatur=off
  Discrete-Time Integrator : DiscreteIntegrator  SampleTime=Ts  ICPrevOutput=DiscIntNeverNeededParam  ICPrevScaledInput=DiscIntNeverNeededParam
  I : Gain  Gain=Ki
  p : Gain  Gain=Kp
  Curcmd(Amp) : Outport
  wires:
  Discrete-Time Integrator/1 -> Add1/2
  Diff/1 -> Add1/3
  D/1 -> Diff/1
  Add1/1 -> Curcmd(Amp)/1
  I/1 -> Discrete-Time Integrator/1
  p/1 -> Add1/1
  Error(LpTs)/1 -> D/1, I/1, p/1

== system CtrPlatform/Controller/Source Model/PosVel Pulse Cmd ==
  Enable : Inport
  Add1 : Sum
  CmdVel(rpm) : Scope
      settings: SaveName=ScopeData2
  Data Type  Conversion : DataTypeConversion  OutDataTypeStr=uint8  SaturateOnIntegerOverflow=on  RndMeth=Zero
  Discrete  2nd-Order Filter : powerlib_extras/Discrete  Control Blocks/Discrete  2nd-Order Filter  FilterType=Lowpass  Fo=10  Zeta=0.9  Ts=Ts_Dyn  Initialize=off  Vac_Init=[0.8 -25 60]  Vdc_Init=-0.4  PlotResponse=off  param1=[1 500 1]
  LinePTs2Rpm : Gain  Gain=LinePTs2Rpm
  Logical Operator : Logic  Operator=NOT  AllPortsSameDT=off  OutDataTypeStr=boolean
  Logical Operator1 : Logic  Operator=OR  AllPortsSameDT=off  OutDataTypeStr=boolean
  Multiport Switch : MultiPortSwitch  Inputs=2  zeroidx=off
  One : Constant  OutDataTypeStr=boolean  SampleTime=Ts_Dyn
  Pulse Generator : Subsystem
  Triggered Subsystem : Subsystem  TreatAsAtomicUnit=on
  Zero Refrence : Subsystem
  Cmd(LpTs) : Outport
  wires:
  LinePTs2Rpm/1 -> CmdVel(rpm)/1
  Logical Operator/1 -> Logical Operator1/1
  Zero Refrence/1(Pulse) -> Multiport Switch/3
  Pulse Generator/1(Pulse(LinePTs)) -> Multiport Switch/2
  One/1 -> Add1/2
  Add1/1 -> Multiport Switch/1
  Data Type  Conversion/1 -> Add1/1
  Multiport Switch/1 -> Discrete  2nd-Order Filter/1
  Enable/1 -> Logical Operator/1, Pulse Generator/Enable
  Logical Operator1/1 -> Data Type  Conversion/1, Zero Refrence/Enable
  Triggered Subsystem/1(Out1) -> Logical Operator1/2
  Discrete  2nd-Order Filter/1 -> LinePTs2Rpm/1, Cmd(LpTs)/1
  Pulse Generator/2(TimePulse) -> Triggered Subsystem/Trigger

== system CtrPlatform/Controller/Source Model/Vel Pulse Cmd ==
  Enable : Inport
  Add1 : Sum
  CmdVel(rpm) : Scope
      settings: SaveName=ScopeData2
  Data Type  Conversion : DataTypeConversion  OutDataTypeStr=uint8  SaturateOnIntegerOverflow=on  RndMeth=Zero
  Discrete  2nd-Order Filter : powerlib_extras/Discrete  Control Blocks/Discrete  2nd-Order Filter  FilterType=Lowpass  Fo=10  Zeta=0.9  Ts=Ts_Dyn  Initialize=off  Vac_Init=[0.8 -25 60]  Vdc_Init=-0.4  PlotResponse=off  param1=[1 500 1]
  LinePTs2Rpm : Gain  Gain=LinePTs2Rpm
  Logical Operator : Logic  Operator=NOT  AllPortsSameDT=off  OutDataTypeStr=boolean
  Logical Operator1 : Logic  Operator=OR  AllPortsSameDT=off  OutDataTypeStr=boolean
  Multiport Switch : MultiPortSwitch  Inputs=2  zeroidx=off
  One : Constant  OutDataTypeStr=boolean  SampleTime=Ts_Dyn
  Pulse Generator : Subsystem
  Triggered Subsystem : Subsystem  TreatAsAtomicUnit=on
  Zero Refrence : Subsystem
  Cmd(LpTs) : Outport
  wires:
  Pulse Generator/2(TimePulse) -> Triggered Subsystem/Trigger
  Discrete  2nd-Order Filter/1 -> Cmd(LpTs)/1, LinePTs2Rpm/1
  Triggered Subsystem/1(Out1) -> Logical Operator1/2
  Logical Operator1/1 -> Zero Refrence/Enable, Data Type  Conversion/1
  Enable/1 -> Pulse Generator/Enable, Logical Operator/1
  Multiport Switch/1 -> Discrete  2nd-Order Filter/1
  Data Type  Conversion/1 -> Add1/1
  Add1/1 -> Multiport Switch/1
  One/1 -> Add1/2
  Pulse Generator/1(Pulse(LinePTs)) -> Multiport Switch/2
  Zero Refrence/1(Pulse) -> Multiport Switch/3
  Logical Operator/1 -> Logical Operator1/1
  LinePTs2Rpm/1 -> CmdVel(rpm)/1

== system CtrPlatform/Display/EndTrjDisplay/EndAccDisplay ==
  EndAcc : Inport
  Ref_EndAcc : Inport  Port=2
  AVx : Scope  NumInputPorts=2
      settings: TimeRange=10  YMin=-2.999999999999999e-017~-1  YMax=4e-017~1
  "AVy " : Scope  NumInputPorts=2
      settings: YMin=-5~-5  YMax=5~5
  AVz : Scope  NumInputPorts=2
      settings: YMin=-5~-5  YMax=5~5  SaveName=ScopeData2
  AWx : Scope  NumInputPorts=2
      settings: YMin=-5~-5  YMax=5~5  SaveName=ScopeData3
  AWy : Scope  NumInputPorts=2
      settings: TimeRange=10  YMin=-4.18~4.060000000000001  YMax=-4.04~4.2  SaveName=ScopeData4
  AWz : Scope  NumInputPorts=2
      settings: TimeRange=10  YMin=-1.6e-006~-0.003  YMax=4e-007~0.004  SaveName=ScopeData5
  Demux : Demux  Outputs=6
  Demux1 : Demux  Outputs=6
  Enc End Acc : ToWorkspace  VariableName=EncEndAcc  SampleTime=-1  SaveFormat=Structure
  Err{1..6} (6 alike) : Scope
      Err1 settings: SaveName=ScopeData6
      Err2 settings: SaveName=ScopeData7
      Err3 settings: SaveName=ScopeData8
      Err4 settings: SaveName=ScopeData9
      Err5 settings: TimeRange=3  YMin=-2.5  YMax=1  SaveName=ScopeData10
      Err6 settings: SaveName=ScopeData11
  Ref End Acc : ToWorkspace  VariableName=RefEndAcc  SampleTime=-1  SaveFormat=Structure
  Sum{,1..5} (6 alike) : Sum  Inputs=+|-
  wires:
  Sum/1 -> Err1/1
  Sum1/1 -> Err2/1
  Sum2/1 -> Err3/1
  Sum3/1 -> Err4/1
  Sum4/1 -> Err5/1
  Sum5/1 -> Err6/1
  EndAcc/1 -> Demux/1, Enc End Acc/1
  Ref_EndAcc/1 -> Demux1/1, Ref End Acc/1
  Demux/1 -> Sum/1, AVx/1
  Demux1/1 -> Sum/2, AVx/2
  Demux/2 -> "AVy "/1, Sum1/1
  Demux/3 -> AVz/1, Sum2/1
  Demux/4 -> Sum3/1, AWx/1
  Demux/5 -> AWy/1, Sum4/1
  Demux/6 -> AWz/1, Sum5/1
  Demux1/2 -> "AVy "/2, Sum1/2
  Demux1/3 -> AVz/2, Sum2/2
  Demux1/4 -> Sum3/2, AWx/2
  Demux1/5 -> AWy/2, Sum4/2
  Demux1/6 -> AWz/2, Sum5/2

== system CtrPlatform/Display/EndTrjDisplay/EndPosDisplay ==
  EndPos : Inport
  Ref_EndPos : Inport  Port=2
  Demux : Demux  Outputs=3
  Demux1 : Demux  Outputs=3
  "Encoder " : ToWorkspace  VariableName=EncEndPos  SampleTime=-1  SaveFormat=Structure
  Err1 : Scope
      settings: SaveName=ScopeData6
  Err2 : Scope
      settings: SaveName=ScopeData7
  Err3 : Scope
      settings: SaveName=ScopeData8
  Mux : Mux  Inputs=2
  Mux1 : Mux  Inputs=2
  Mux2 : Mux  Inputs=2
  "Ref " : ToWorkspace  VariableName=RefEndPos  SampleTime=-1  SaveFormat=Structure
  Sum : Sum  Inputs=+|-
  Sum1 : Sum  Inputs=+|-
  Sum2 : Sum  Inputs=+|-
  X : Scope
      settings: TimeRange=5  YMin=1166  YMax=1166  SaveName=EndPosX
  "Y " : Scope
      settings: YMin=5  YMax=55  SaveName=EndPosY
  Z : Scope
      settings: SaveName=EndPosZ
  wires:
  Ref_EndPos/1 -> "Ref "/1, Demux1/1
  EndPos/1 -> "Encoder "/1, Demux/1
  Sum2/1 -> Err3/1
  Sum1/1 -> Err2/1
  Sum/1 -> Err1/1
  Demux/1 -> Sum/1, Mux/1
  Demux1/1 -> Sum/2, Mux/2
  Demux/2 -> Sum1/1, Mux1/1
  Demux1/2 -> Sum1/2, Mux1/2
  Demux/3 -> Sum2/1, Mux2/1
  Demux1/3 -> Sum2/2, Mux2/2
  Mux/1 -> X/1
  Mux1/1 -> "Y "/1
  Mux2/1 -> Z/1

== system CtrPlatform/Display/EndTrjDisplay/EndVelDisplay ==
  note: Vz
  EndVel : Inport
  Ref_EndVel : Inport  Port=2
  Demux : Demux  Outputs=6
  Demux1 : Demux  Outputs=6
  Enc End Vel : ToWorkspace  VariableName=EncEndVel  SampleTime=-1  SaveFormat=Structure
  Err{1..6} (6 alike) : Scope
      Err1 settings: SaveName=ScopeData6
      Err2 settings: SaveName=ScopeData7
      Err3 settings: SaveName=ScopeData8
      Err4 settings: SaveName=ScopeData9
      Err5 settings: TimeRange=3  YMin=-2.5  YMax=1  SaveName=ScopeData10
      Err6 settings: SaveName=ScopeData11
  R3 : Scope  NumInputPorts=2
      settings: YMin=-5~-5  YMax=5~5  SaveName=ScopeData2
  Ref End Vel : ToWorkspace  VariableName=RefEndVel  SampleTime=-1  SaveFormat=Structure
  Sum{,1..5} (6 alike) : Sum  Inputs=+|-
  Vx : Scope  NumInputPorts=2
      settings: TimeRange=1  YMin=-400~-1  YMax=1200~1
  "Vy " : Scope  NumInputPorts=2
      settings: YMin=-5~-5  YMax=5~5
  Wx : Scope  NumInputPorts=2
      settings: YMin=-5~-5  YMax=5~5  SaveName=ScopeData3
  Wy : Scope  NumInputPorts=2
      settings: TimeRange=10  YMin=-4.18~4.060000000000001  YMax=-4.04~4.2  SaveName=ScopeData4
  Wz : Scope  NumInputPorts=2
      settings: TimeRange=10  YMin=-1.6e-006~-0.003  YMax=4e-007~0.004  SaveName=ScopeData5
  wires:
  Demux1/6 -> Sum5/2, Wz/2
  Demux1/5 -> Sum4/2, Wy/2
  Demux1/4 -> Wx/2, Sum3/2
  Demux1/3 -> Sum2/2, R3/2
  Demux1/2 -> Sum1/2, "Vy "/2
  Demux/6 -> Sum5/1, Wz/1
  Demux/5 -> Sum4/1, Wy/1
  Demux/4 -> Wx/1, Sum3/1
  Demux/3 -> Sum2/1, R3/1
  Demux/2 -> Sum1/1, "Vy "/1
  Demux1/1 -> Vx/2, Sum/2
  Demux/1 -> Vx/1, Sum/1
  Ref_EndVel/1 -> Ref End Vel/1, Demux1/1
  EndVel/1 -> Enc End Vel/1, Demux/1
  Sum5/1 -> Err6/1
  Sum4/1 -> Err5/1
  Sum3/1 -> Err4/1
  Sum2/1 -> Err3/1
  Sum1/1 -> Err2/1
  Sum/1 -> Err1/1

== system CtrPlatform/Display/JntVelAccDisplay/Joint1 ==
  JVA1 : Inport
  Ref_JVA1 : Inport  Port=2
  Acceleration : Scope
      settings: YMin=-5.76  YMax=-5.69  SaveName=ScopeData54
  Angle : Scope
      settings: TimeRange=8  YMin=8.025  YMax=8.575  SaveName=ScopeData52
  Demux : Demux  Outputs=3
  Demux1 : Demux  Outputs=3
  "Encoder " : ToWorkspace  VariableName=EncJVAJ1  SampleTime=-1  SaveFormat=Structure
  Err1 : Scope
      settings: SaveName=ScopeData6
  Err2 : Scope
      settings: SaveName=ScopeData7
  Err3 : Scope
      settings: SaveName=ScopeData8
  Mux : Mux  Inputs=2
  Mux1 : Mux  Inputs=2
  Mux2 : Mux  Inputs=2
  "Ref " : ToWorkspace  VariableName=RefJVAJ1  SampleTime=-1  SaveFormat=Structure
  Sum : Sum  Inputs=+|-
  Sum1 : Sum  Inputs=+|-
  Sum2 : Sum  Inputs=+|-
  "Velocity " : Scope
      settings: YMin=0.35  YMax=1.05  SaveName=ScopeData53
  wires:
  Ref_JVA1/1 -> "Ref "/1, Demux1/1
  JVA1/1 -> "Encoder "/1, Demux/1
  Sum2/1 -> Err3/1
  Sum1/1 -> Err2/1
  Sum/1 -> Err1/1
  Demux/1 -> Sum/1, Mux/1
  Demux1/1 -> Sum/2, Mux/2
  Demux/2 -> Sum1/1, Mux1/1
  Demux1/2 -> Sum1/2, Mux1/2
  Demux/3 -> Sum2/1, Mux2/1
  Demux1/3 -> Sum2/2, Mux2/2
  Mux/1 -> Angle/1
  Mux1/1 -> "Velocity "/1
  Mux2/1 -> Acceleration/1

== system CtrPlatform/Display/JntVelAccDisplay/Joint2 ==
  JVA2 : Inport
  Ref_JVA2 : Inport  Port=2
  Acceleration : Scope  NumInputPorts=2
      settings: YMin=0.0255~-0.599  YMax=0.03125~-0.581  SaveName=ScopeData2
  Angle : Scope  NumInputPorts=2
      settings: YMin=-9.5~-0.3  YMax=-6.5~-0.225
  Demux : Demux  Outputs=3
  Demux1 : Demux  Outputs=3
  "Encoder " : ToWorkspace  VariableName=EncJVAJ2  SampleTime=-1  SaveFormat=Structure
  Err1 : Scope
      settings: SaveName=ScopeData6
  Err2 : Scope
      settings: SaveName=ScopeData7
  Err3 : Scope
      settings: SaveName=ScopeData8
  "Ref " : ToWorkspace  VariableName=RefJVAJ2  SampleTime=-1  SaveFormat=Structure
  Sum : Sum  Inputs=+|-
  Sum1 : Sum  Inputs=+|-
  Sum2 : Sum  Inputs=+|-
  "Velocity " : Scope  NumInputPorts=2
      settings: YMin=0.00875~0.17  YMax=0.0097~0.205
  wires:
  Demux1/3 -> Sum2/2, Acceleration/2
  Demux/3 -> Sum2/1, Acceleration/1
  Demux1/2 -> Sum1/2, "Velocity "/2
  Demux/2 -> Sum1/1, "Velocity "/1
  Demux1/1 -> Sum/2, Angle/2
  Demux/1 -> Sum/1, Angle/1
  Sum/1 -> Err1/1
  Sum1/1 -> Err2/1
  Sum2/1 -> Err3/1
  JVA2/1 -> Demux/1, "Encoder "/1
  Ref_JVA2/1 -> Demux1/1, "Ref "/1

== system CtrPlatform/Display/JntVelAccDisplay/Joint3 ==
  JVA3 : Inport
  Ref_JVA3 : Inport  Port=2
  Acceleration : Scope  NumInputPorts=2
      settings: YMin=-5~-5  YMax=5~5  SaveName=ScopeData2
  Angle : Scope  NumInputPorts=2
      settings: TimeRange=10  YMin=-2.999999999999999e-017~-1  YMax=4e-017~1
  Demux : Demux  Outputs=3
  Demux1 : Demux  Outputs=3
  "Encoder " : ToWorkspace  VariableName=EncJVAJ3  SampleTime=-1  SaveFormat=Structure
  Err1 : Scope
      settings: SaveName=ScopeData6
  Err2 : Scope
      settings: SaveName=ScopeData7
  Err3 : Scope
      settings: SaveName=ScopeData8
  "Ref " : ToWorkspace  VariableName=RefJVAJ3  SampleTime=-1  SaveFormat=Structure
  Sum : Sum  Inputs=+|-
  Sum1 : Sum  Inputs=+|-
  Sum2 : Sum  Inputs=+|-
  "Velocity " : Scope  NumInputPorts=2
      settings: YMin=-5~-5  YMax=5~5
  wires:
  Ref_JVA3/1 -> "Ref "/1, Demux1/1
  JVA3/1 -> "Encoder "/1, Demux/1
  Sum2/1 -> Err3/1
  Sum1/1 -> Err2/1
  Sum/1 -> Err1/1
  Demux/1 -> Angle/1, Sum/1
  Demux1/1 -> Angle/2, Sum/2
  Demux/2 -> "Velocity "/1, Sum1/1
  Demux1/2 -> "Velocity "/2, Sum1/2
  Demux/3 -> Acceleration/1, Sum2/1
  Demux1/3 -> Acceleration/2, Sum2/2
